simulink model "prescan_repl_stop_cam_radar"  (R2019a)
settings: Solver=VariableStepAuto  StartTime=0.0  StopTime=100  RelTol=1e-3
libraries: ProSivic_Sensors x4, simulink x1, realtime_pacer_lib x1
settings Model: Creator=Markus Borg  LastModifiedBy=Markus Borg

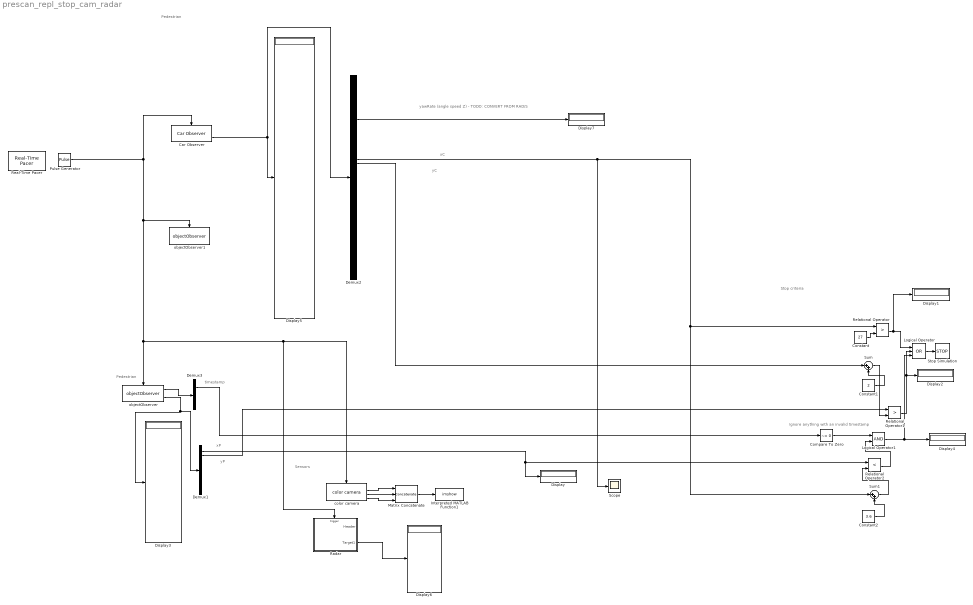
== system prescan_repl_stop_cam_radar ==
  note: Stop criteria
  note: yP
  note: yC
  note: xP
  note: xC
  note: Pedestrian
  note: Sensors
  note: Pedestrian
  note: yawRate (angle speed Z) - TODO: CONVERT FROM RAD/S
  note: timestamp
  note: Ignore anything with an invalid timestamp
  " color camera" : ProSivic_Sensors/ color camera  topic=dashcam/cam  h=375  w=500  color=on
  Car Observer : ProSivic_Sensors/Car Observer  SystemSampleTime=-1
      link override S-Function: topic=egocar_obs/car_obs
  Compare To Zero : simulink/Logic and Bit Operations/Compare To Zero  relop=~=  OutDataTypeStr=boolean
  Constant : Constant  Value=27
  Constant1 : Constant  Value=2
  Constant2 : Constant  Value=3.6
  Demux1 : Demux  Outputs=10
  Demux2 : Demux  Outputs=40
  Demux3 : Demux  Outputs=2
  Display{,1..7} (8 alike) : Display
  Interpreted MATLAB Function1 : MATLABFcn  MATLABFcn=imshow  OutputDimensions=0
  Logical Operator : Logic  Operator=OR  Inputs=3  AllPortsSameDT=off  OutDataTypeStr=boolean
  Logical Operator1 : Logic  AllPortsSameDT=off  OutDataTypeStr=boolean
  Matrix Concatenate : Concatenate  NumInputs=3  Mode=Multidimensional array  ConcatenateDimension=2
  Pulse Generator : DiscretePulseGenerator  PulseType=Time based  Period=0.005  PulseWidth=50
  Radar : Subsystem  Description=Radar block retreives the latest radar information from the ProSiVIC DDS store.  AncestorBlock=ProSivic_Sensors/Radar  TreatAsAtomicUnit=on
  Real-Time Pacer : realtime_pacer_lib/Real-Time Pacer  simTimePerRealTime=10
  Relational Operator : RelationalOperator  Operator=>  OutDataTypeStr=boolean  RndMeth=Simplest
  Relational Operator1 : RelationalOperator  Operator=>  OutDataTypeStr=boolean  RndMeth=Simplest
  Relational Operator2 : RelationalOperator  Operator=<  OutDataTypeStr=boolean  RndMeth=Simplest
  Scope : Scope
  Stop Simulation : Stop
  Sum : Sum  Inputs=|++
  Sum1 : Sum  Inputs=|++
  objectObserver : ProSivic_Sensors/objectObserver  topic=ped_obs
  objectObserver1 : ProSivic_Sensors/objectObserver  topic=car_obj_obs
  wires:
  Pulse Generator/1 -> objectObserver/Trigger, Radar/Trigger, " color camera"/Trigger, objectObserver1/Trigger, Car Observer/Trigger
  Relational Operator1/1 -> Display2/1, Logical Operator/2
  Demux1/1 -> Relational Operator2/1, Display/1
  Constant/1 -> Relational Operator/2
  objectObserver/2 -> Display3/1, Demux1/1
  Relational Operator/1 -> Display1/1, Logical Operator/1
  Constant1/1 -> Sum/2
  Demux1/2 -> Relational Operator1/1
  Constant2/1 -> Sum1/2
  Sum1/1 -> Relational Operator2/2
  Sum/1 -> Relational Operator1/2
  Logical Operator/1 -> Stop Simulation/1
  " color camera"/4 -> Matrix Concatenate/3
  " color camera"/3 -> Matrix Concatenate/2
  Matrix Concatenate/1 -> Interpreted MATLAB Function1/1
  " color camera"/2 -> Matrix Concatenate/1
  Car Observer/2 -> Demux2/1, Display5/1
  Radar/2(Target1) -> Display6/1
  Demux2/16 -> Scope/1, Sum1/1, Relational Operator/1
  Demux2/17 -> Sum/1
  Demux2/6 -> Display7/1
  objectObserver/1 -> Demux3/1
  Demux3/1 -> Compare To Zero/1
  Compare To Zero/1 -> Logical Operator1/1
  Relational Operator2/1 -> Logical Operator1/2
  Logical Operator1/1 -> Logical Operator/3, Display4/1

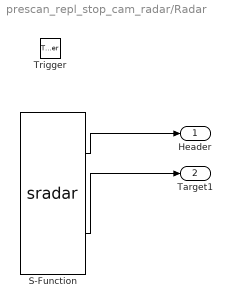
== system prescan_repl_stop_cam_radar/Radar ==
  Trigger : TriggerPort  VariantControl=Variant
  S-Function : S-Function  FunctionName=sradar  Parameters=topic,nbmaxtarget  SFunctionDeploymentMode=off  EnableBusSupport=off  mask{topic=radar/radar, nbmaxtarget=1}
      mask prompts: topic "Radar Name"; nbmaxtarget "Number of targets"
  Header : Outport
  Target1 : Outport  Port=2
  wires:
  S-Function/2 -> Target1/1
  S-Function/1 -> Header/1
